simulink model "ICAR"  (R2018b)
settings: Solver=FixedStepAuto  StartTime=0.0  StopTime=10.0  RelTol=1e-3
(part 2 of 4)

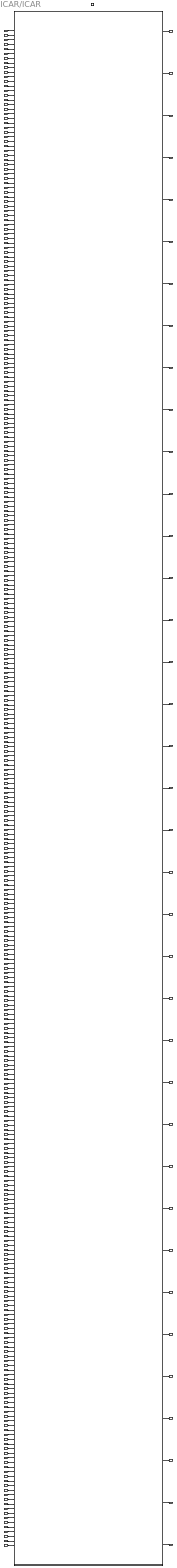
== system ICAR/ICAR ==
  System_Clock : Inport  OutDataTypeStr=UInt16
  FDMMve_d_IcaFcnConf : Inport  Port=2  OutDataTypeStr=UInt16
  FDMMve_d_SignalTStamp : Inport  Port=3  OutDataTypeStr=UInt16
  ICABva_g_VehParameter : Inport  Port=4  OutDataTypeStr=T_M_Nm_Float32  PortDimensions=60
  ICABva_g_FilterInfo : Inport  Port=5  OutDataTypeStr=T_M_Nm_Float32  PortDimensions=50
  ICABve_d_SignalTStamp : Inport  Port=6  OutDataTypeStr=UInt16
  IMAPve_d_EPS_LKA_State : Inport  Port=7  OutDataTypeStr=UInt16
  IMAPve_g_EPS_SW_Trq : Inport  Port=8  OutDataTypeStr=T_M_Nm_Float32
  IMAPve_d_EPS_Error_State : Inport  Port=9  OutDataTypeStr=UInt16
  IMAPve_d_EPS_Trq_State : Inport  Port=10  OutDataTypeStr=UInt16
  IMAPve_d_SAS_Clb_State : Inport  Port=11  OutDataTypeStr=UInt16
  IMAPve_d_SAS_Trim_State : Inport  Port=12  OutDataTypeStr=UInt16
  IMAPve_d_EPS_TrqLim_State : Inport  Port=13  OutDataTypeStr=UInt16
  IMAPve_g_EPS_LKA_Current : Inport  Port=14  OutDataTypeStr=T_M_Nm_Float32
  IMAPve_g_ESC_LatAcc : Inport  Port=15  OutDataTypeStr=T_M_Nm_Float32
  IMAPve_d_ESC_LatAcc_Valid : Inport  Port=16  OutDataTypeStr=UInt16
  IMAPve_g_ESC_YawRate : Inport  Port=17  OutDataTypeStr=T_M_Nm_Float32
  IMAPve_d_ESC_YawRate_Valid : Inport  Port=18  OutDataTypeStr=UInt16
  IMAPve_g_ESC_UnYawRate : Inport  Port=19  OutDataTypeStr=T_M_Nm_Float32
  IMAPve_g_ESC_VehSpd : Inport  Port=20  OutDataTypeStr=T_M_Nm_Float32
  IMAPve_g_ESC_LonAcc : Inport  Port=21  OutDataTypeStr=T_M_Nm_Float32
  IMAPve_d_ESC_LonAcc_Valid : Inport  Port=22  OutDataTypeStr=UInt16
  IMAPve_g_ESC_Brake_Press : Inport  Port=23  OutDataTypeStr=T_M_Nm_Float32
  IMAPve_g_ESC_Static_Slope : Inport  Port=24  OutDataTypeStr=T_M_Nm_Float32
  IMAPve_g_ESC_DySlope_Accuracy : Inport  Port=25  OutDataTypeStr=T_M_Nm_Float32
  IMAPve_g_ESC_DySlope : Inport  Port=26  OutDataTypeStr=T_M_Nm_Float32
  IMAPve_g_SW_Angle : Inport  Port=27  OutDataTypeStr=T_M_Nm_Float32
  IMAPve_g_SW_Angle_Speed : Inport  Port=28  OutDataTypeStr=T_M_Nm_Float32
  IMAPve_d_BCM_HazardLamp : Inport  Port=29  OutDataTypeStr=UInt16
  IMAPve_d_BCM_Left_Light : Inport  Port=30  OutDataTypeStr=UInt16
  IMAPve_d_BCM_Right_Light : Inport  Port=31  OutDataTypeStr=UInt16
  IMAPve_d_ESC_BrakeLamp_Req : Inport  Port=32  OutDataTypeStr=UInt16
  IMAPve_d_BCM_Opening_State : Inport  Port=33  OutDataTypeStr=UInt16
  IMAPve_d_BCM_Trunk_State : Inport  Port=34  OutDataTypeStr=UInt16
  IMAPve_d_BCM_LF_Door_State : Inport  Port=35  OutDataTypeStr=UInt16
  IMAPve_d_BCM_RF_Door_State : Inport  Port=36  OutDataTypeStr=UInt16
  IMAPve_d_BCM_RR_Door_State : Inport  Port=37  OutDataTypeStr=UInt16
  IMAPve_d_BCM_LR_Door_State : Inport  Port=38  OutDataTypeStr=UInt16
  IMAPve_d_SCC_Left_SwitchSig : Inport  Port=39  OutDataTypeStr=UInt16
  IMAPve_d_SCC_Right_SwitchSig : Inport  Port=40  OutDataTypeStr=UInt16
  IMAPve_d_PEPS_Door_Lock_Req : Inport  Port=41  OutDataTypeStr=UInt16
  IMAPve_d_BCM_Door_Lock_State : Inport  Port=42  OutDataTypeStr=UInt16
  IMAPve_d_EMS_ACC_Status : Inport  Port=43  OutDataTypeStr=UInt16
  IMAPve_g_EMS_Pot_WhlT_Max : Inport  Port=44  OutDataTypeStr=T_M_Nm_Float32
  IMAPve_g_EMS_Pot_WhlT_Min : Inport  Port=45  OutDataTypeStr=T_M_Nm_Float32
  IMAPve_g_EMS_RealPedal : Inport  Port=46  OutDataTypeStr=T_M_Nm_Float32
  IMAPve_g_EMS_MaxTWhl : Inport  Port=47  OutDataTypeStr=T_M_Nm_Float32
  IMAPve_g_EMS_MaxTWhl_Offset : Inport  Port=48  OutDataTypeStr=T_M_Nm_Float32
  IMAPve_g_EMS_MinTWhl : Inport  Port=49  OutDataTypeStr=T_M_Nm_Float32
  IMAPve_g_EMS_MinTWhl_Offset : Inport  Port=50  OutDataTypeStr=T_M_Nm_Float32
  IMAPve_g_EMS_Actual_FlwT : Inport  Port=51  OutDataTypeStr=T_M_Nm_Float32
  IMAPve_g_EMS_Actual_IndT : Inport  Port=52  OutDataTypeStr=T_M_Nm_Float32
  IMAPve_g_EMS_Realize_TWhl : Inport  Port=53  OutDataTypeStr=T_M_Nm_Float32
  IMAPve_g_EMS_ACC_VirtualPedal : Inport  Port=54  OutDataTypeStr=T_M_Nm_Float32
  IMAPve_d_EMS_AccPedal_Fault : Inport  Port=55  OutDataTypeStr=UInt16
  IMAPve_g_EMS_Driver_Torque : Inport  Port=56  OutDataTypeStr=T_M_Nm_Float32
  IMAPve_d_ESC_Brake_Effort : Inport  Port=57  OutDataTypeStr=UInt16
  IMAPve_g_EMS_Engine_Speed : Inport  Port=58  OutDataTypeStr=T_M_Nm_Float32
  IMAPve_d_ESC_Veh_Standstill : Inport  Port=59  OutDataTypeStr=UInt16
  IMAPve_d_TCU_Actual_Gear : Inport  Port=60  OutDataTypeStr=UInt16
  IMAPve_d_TCU_Target_Gear : Inport  Port=61  OutDataTypeStr=UInt16
  IMAPve_d_TCU_PRND_State : Inport  Port=62  OutDataTypeStr=UInt16
  IMAPve_d_BCM_Ignition_State : Inport  Port=63  OutDataTypeStr=UInt16
  IMAPve_d_ACU_Driver_Belt : Inport  Port=64  OutDataTypeStr=UInt16
  IMAPve_d_SWS_Fault_Code : Inport  Port=65  OutDataTypeStr=UInt16
  IMAPve_d_SWS_Failure_Status : Inport  Port=66  OutDataTypeStr=UInt16
  IMAPve_d_ESC_OFF : Inport  Port=67  OutDataTypeStr=UInt16
  IMAPve_d_ESC_AlarmSig : Inport  Port=68  OutDataTypeStr=UInt16
  IMAPve_d_Speed_Limit_Switch : Inport  Port=69  OutDataTypeStr=UInt16
  IMAPve_d_ESC_ESC_Active : Inport  Port=70  OutDataTypeStr=UInt16
  IMAPve_d_ESC_MSR_Active : Inport  Port=71  OutDataTypeStr=UInt16
  IMAPve_d_ESC_TCS_Active : Inport  Port=72  OutDataTypeStr=UInt16
  IMAPve_d_ESC_VehSpd_Valid : Inport  Port=73  OutDataTypeStr=UInt16
  IMAPve_d_Brake_Pedal_Fault : Inport  Port=74  OutDataTypeStr=UInt16
  IMAPve_d_ESC_ABS_Active : Inport  Port=75  OutDataTypeStr=UInt16
  IMAPve_d_ESC_ABS_Valid : Inport  Port=76  OutDataTypeStr=UInt16
  IMAPve_d_ESC_ABS_AlarmSig : Inport  Port=77  OutDataTypeStr=UInt16
  IMAPve_d_ESC_FL_WheelPulVal : Inport  Port=78  OutDataTypeStr=UInt16
  IMAPve_d_ESC_FR_WheelPulVal : Inport  Port=79  OutDataTypeStr=UInt16
  IMAPve_d_ESC_RL_WheelPulVal : Inport  Port=80  OutDataTypeStr=UInt16
  IMAPve_d_ESC_RR_WheelPulVal : Inport  Port=81  OutDataTypeStr=UInt16
  IMAPve_g_ESC_FL_WhlSpd : Inport  Port=82  OutDataTypeStr=T_M_Nm_Float32
  IMAPve_d_ESC_FL_WhlSpd_Fault : Inport  Port=83  OutDataTypeStr=UInt16
  IMAPve_g_ESC_FR_WhlSpd : Inport  Port=84  OutDataTypeStr=T_M_Nm_Float32
  IMAPve_d_ESC_FR_WhlSpd_Fault : Inport  Port=85  OutDataTypeStr=UInt16
  IMAPve_g_ESC_RL_WhlSpd : Inport  Port=86  OutDataTypeStr=T_M_Nm_Float32
  IMAPve_d_ESC_RL_WhlSpd_Fault : Inport  Port=87  OutDataTypeStr=UInt16
  IMAPve_g_ESC_RR_WhlSpd : Inport  Port=88  OutDataTypeStr=T_M_Nm_Float32
  IMAPve_d_ESC_RR_WhlSpd_Fault : Inport  Port=89  OutDataTypeStr=UInt16
  IMAPve_d_ESC_FL_Wheel_Pulse : Inport  Port=90  OutDataTypeStr=UInt16
  IMAPve_d_ESC_FR_Wheel_Pulse : Inport  Port=91  OutDataTypeStr=UInt16
  IMAPve_d_ESC_RL_Wheel_Pulse : Inport  Port=92  OutDataTypeStr=UInt16
  IMAPve_d_ESC_RR_Wheel_Pulse : Inport  Port=93  OutDataTypeStr=UInt16
  IMAPve_d_TCU_AT_Failure : Inport  Port=94  OutDataTypeStr=UInt16
  IMAPve_d_TCU_Shift_Valid : Inport  Port=95  OutDataTypeStr=UInt16
  IMAPve_d_TCU_DCT_Clutch_State : Inport  Port=96  OutDataTypeStr=UInt16
  IMAPve_d_TCU_Gear_Engage : Inport  Port=97  OutDataTypeStr=UInt16
  IMAPve_d_TCU_Select_ATMode : Inport  Port=98  OutDataTypeStr=UInt16
  IMAPve_d_EMS_Engine_Status : Inport  Port=99  OutDataTypeStr=UInt16
  IMAPve_d_EMS_Gearbox_CtlAvail : Inport  Port=100  OutDataTypeStr=UInt16
  IMAPve_d_ESC_Brake_Failsafe : Inport  Port=101  OutDataTypeStr=UInt16
  IMAPve_d_ESC_AEB_Status : Inport  Port=102  OutDataTypeStr=UInt16
  IMAPve_d_ESC_AEB_Available : Inport  Port=103  OutDataTypeStr=UInt16
  IMAPve_d_ESC_AEB_Active : Inport  Port=104  OutDataTypeStr=UInt16
  IMAPve_d_ESC_ACC_Status : Inport  Port=105  OutDataTypeStr=UInt16
  IMAPve_d_ESC_ACC_Available : Inport  Port=106  OutDataTypeStr=UInt16
  IMAPve_d_ESC_ACC_Active : Inport  Port=107  OutDataTypeStr=UInt16
  IMAPve_d_EMS_ACC_Effective : Inport  Port=108  OutDataTypeStr=UInt16
  IMAPve_d_BCM_FrontWiper_State : Inport  Port=109  OutDataTypeStr=UInt16
  IMAPve_d_BCM_CHMSL_Status : Inport  Port=110  OutDataTypeStr=UInt16
  IMAPve_d_BCM_BrakeLamp_State : Inport  Port=111  OutDataTypeStr=UInt16
  IMAPve_d_GW_Brake_Only_Req : Inport  Port=112  OutDataTypeStr=UInt16
  IMAPve_d_ACU_Passenger_Belt : Inport  Port=113  OutDataTypeStr=UInt16
  IMAPve_d_EMS_ACC_CtlAvail : Inport  Port=114  OutDataTypeStr=UInt16
  IMAPve_d_EMS_ACC_Inhibited : Inport  Port=115  OutDataTypeStr=UInt16
  IMAPve_d_EMS_Brake_Pedal : Inport  Port=116  OutDataTypeStr=UInt16
  IMAPve_d_BCM_LowBeam_State : Inport  Port=117  OutDataTypeStr=UInt16
  IMAPve_d_BCM_HighBeam_State : Inport  Port=118  OutDataTypeStr=UInt16
  IMAPve_d_EPB_Status : Inport  Port=119  OutDataTypeStr=UInt16
  IMAPve_d_EPB_Display_Req : Inport  Port=120  OutDataTypeStr=UInt16
  IMAPve_d_EPB_Warn_Req : Inport  Port=121  OutDataTypeStr=UInt16
  IMAPve_d_EPB_Switch_State : Inport  Port=122  OutDataTypeStr=UInt16
  IMAPve_d_EPB_Switch_Valid : Inport  Port=123  OutDataTypeStr=UInt16
  IMAPve_d_ESC_Drive_Direction : Inport  Port=124  OutDataTypeStr=UInt16
  IMAPve_d_ESC_Hold_State : Inport  Port=125  OutDataTypeStr=UInt16
  IMAPve_d_EPS_Steer_Hold_State : Inport  Port=126  OutDataTypeStr=UInt16
  IMAPve_d_EPS_Warning_State : Inport  Port=127  OutDataTypeStr=UInt16
  IMAPve_g_EPS_PowerCon : Inport  Port=128  OutDataTypeStr=T_M_Nm_Float32
  IMAPve_d_ESC_EBD_AlarmSig : Inport  Port=129  OutDataTypeStr=UInt16
  IMAPve_d_ESC_AVH_Status : Inport  Port=130  OutDataTypeStr=UInt16
  IMAPve_d_Radar_Detective_Req : Inport  Port=131  OutDataTypeStr=UInt16
  IMAPve_g_BCM_Battery_Voltage : Inport  Port=132  OutDataTypeStr=T_M_Nm_Float32
  IMAPve_d_TBOX_LocalTimeY : Inport  Port=133  OutDataTypeStr=UInt16
  IMAPve_d_TBOX_LocalTimeM : Inport  Port=134  OutDataTypeStr=UInt16
  IMAPve_d_TBOX_LocalTimeD : Inport  Port=135  OutDataTypeStr=UInt16
  IMAPve_d_TBOX_LocalTimeH : Inport  Port=136  OutDataTypeStr=UInt16
  IMAPve_d_TBOX_LocalTimeMin : Inport  Port=137  OutDataTypeStr=UInt16
  IMAPve_d_TBOX_LocalTimeS : Inport  Port=138  OutDataTypeStr=UInt16
  IMAPve_d_TBOX_LocalTime_Valid : Inport  Port=139  OutDataTypeStr=UInt16
  IMAPve_d_TPMS_Warn_Indicate : Inport  Port=140  OutDataTypeStr=UInt16
  IMAPve_d_Radar_State : Inport  Port=141  OutDataTypeStr=UInt16
  IMAPve_d_ACC_Desired_Headway : Inport  Port=142  OutDataTypeStr=UInt16
  IMAPve_d_Time_System_Clock : Inport  Port=143  OutDataTypeStr=UInt16
  IMAPve_d_Signal_Time_Stamp : Inport  Port=144  OutDataTypeStr=UInt16
  IMAPve_g_GW_IC_Odometer : Inport  Port=145  OutDataTypeStr=UInt32
  IMAPve_g_FAPA_State : Inport  Port=146  OutDataTypeStr=UInt32
  IMAPve_d_Outside_Temp : Inport  Port=147  OutDataTypeStr=UInt16
  IMAPve_d_ORI_CIPV_ID : Inport  Port=148  OutDataTypeStr=UInt16
  IMAPve_d_ORI_Obj_Num : Inport  Port=149  OutDataTypeStr=UInt16
  IMAPva_g_ORI_Probability : Inport  Port=150  OutDataTypeStr=T_M_Nm_Float32  PortDimensions=16
  IMAPva_d_ORI_Obj_Class : Inport  Port=151  OutDataTypeStr=UInt16  PortDimensions=16
  IMAPva_d_ORI_Obj_Motion : Inport  Port=152  OutDataTypeStr=UInt16  PortDimensions=16
  IMAPva_g_ORI_Obj_RelVel : Inport  Port=153  OutDataTypeStr=T_M_Nm_Float32  PortDimensions=16
  IMAPva_g_ORI_Obj_LongDis : Inport  Port=154  OutDataTypeStr=T_M_Nm_Float32  PortDimensions=16
  IMAPva_d_ORI_Obj_Lane : Inport  Port=155  OutDataTypeStr=UInt16  PortDimensions=16
  IMAPva_g_ORI_Obj_LAngle : Inport  Port=156  OutDataTypeStr=T_M_Nm_Float32  PortDimensions=16
  IMAPva_g_ORI_Obj_RAngle : Inport  Port=157  OutDataTypeStr=T_M_Nm_Float32  PortDimensions=16
  IMAPva_g_ORI_Obj_Width : Inport  Port=158  OutDataTypeStr=T_M_Nm_Float32  PortDimensions=16
  IMAPva_d_ORI_Obj_ID : Inport  Port=159  OutDataTypeStr=UInt16  PortDimensions=16
  IMAPve_d_ORI_Lane_Valid : Inport  Port=160  OutDataTypeStr=UInt16
  IMAPve_d_ORI_Lane_ConsArea : Inport  Port=161  OutDataTypeStr=UInt16
  IMAPve_d_ORI_Lane_RoadType : Inport  Port=162  OutDataTypeStr=UInt16
  IMAPve_g_ORI_L0_C3 : Inport  Port=163  OutDataTypeStr=T_M_Nm_Float32
  IMAPve_g_ORI_L0_C2 : Inport  Port=164  OutDataTypeStr=T_M_Nm_Float32
  IMAPve_g_ORI_L0_C1 : Inport  Port=165  OutDataTypeStr=T_M_Nm_Float32
  IMAPve_g_ORI_L0_C0 : Inport  Port=166  OutDataTypeStr=T_M_Nm_Float32
  IMAPve_d_ORI_L0_Q : Inport  Port=167  OutDataTypeStr=UInt16
  IMAPve_d_ORI_L0_Type : Inport  Port=168  OutDataTypeStr=UInt16
  IMAPve_g_ORI_L0_VR : Inport  Port=169  OutDataTypeStr=T_M_Nm_Float32
  IMAPve_g_ORI_L0_TLC : Inport  Port=170  OutDataTypeStr=T_M_Nm_Float32
  IMAPve_g_ORI_L0_W : Inport  Port=171  OutDataTypeStr=T_M_Nm_Float32
  IMAPve_d_ORI_L0_LC : Inport  Port=172  OutDataTypeStr=UInt16
  IMAPve_g_ORI_L1_C3 : Inport  Port=173  OutDataTypeStr=T_M_Nm_Float32
  IMAPve_g_ORI_L1_C2 : Inport  Port=174  OutDataTypeStr=T_M_Nm_Float32
  IMAPve_g_ORI_L1_C1 : Inport  Port=175  OutDataTypeStr=T_M_Nm_Float32
  IMAPve_g_ORI_L1_C0 : Inport  Port=176  OutDataTypeStr=T_M_Nm_Float32
  IMAPve_d_ORI_L1_Q : Inport  Port=177  OutDataTypeStr=UInt16
  IMAPve_d_ORI_L1_Type : Inport  Port=178  OutDataTypeStr=UInt16
  IMAPve_g_ORI_L1_VR : Inport  Port=179  OutDataTypeStr=T_M_Nm_Float32
  IMAPve_g_ORI_L1_TLC : Inport  Port=180  OutDataTypeStr=T_M_Nm_Float32
  IMAPve_g_ORI_L1_W : Inport  Port=181  OutDataTypeStr=T_M_Nm_Float32
  IMAPve_d_ORI_L1_LC : Inport  Port=182  OutDataTypeStr=UInt16
  IMAPve_g_ORI_R0_C3 : Inport  Port=183  OutDataTypeStr=T_M_Nm_Float32
  IMAPve_g_ORI_R0_C2 : Inport  Port=184  OutDataTypeStr=T_M_Nm_Float32
  IMAPve_g_ORI_R0_C1 : Inport  Port=185  OutDataTypeStr=T_M_Nm_Float32
  IMAPve_g_ORI_R0_C0 : Inport  Port=186  OutDataTypeStr=T_M_Nm_Float32
  IMAPve_d_ORI_R0_Q : Inport  Port=187  OutDataTypeStr=UInt16
  IMAPve_d_ORI_R0_LT : Inport  Port=188  OutDataTypeStr=UInt16
  IMAPve_g_ORI_R0_VR : Inport  Port=189  OutDataTypeStr=T_M_Nm_Float32
  IMAPve_g_ORI_R0_TLC : Inport  Port=190  OutDataTypeStr=T_M_Nm_Float32
  IMAPve_g_ORI_R0_W : Inport  Port=191  OutDataTypeStr=T_M_Nm_Float32
  IMAPve_d_ORI_R0_LC : Inport  Port=192  OutDataTypeStr=UInt16
  IMAPve_g_ORI_R1_C3 : Inport  Port=193  OutDataTypeStr=T_M_Nm_Float32
  IMAPve_g_ORI_R1_C2 : Inport  Port=194  OutDataTypeStr=T_M_Nm_Float32
  IMAPve_g_ORI_R1_C1 : Inport  Port=195  OutDataTypeStr=T_M_Nm_Float32
  IMAPve_g_ORI_R1_C0 : Inport  Port=196  OutDataTypeStr=T_M_Nm_Float32
  IMAPve_d_ORI_R1_Q : Inport  Port=197  OutDataTypeStr=UInt16
  IMAPve_d_ORI_R1_LT : Inport  Port=198  OutDataTypeStr=UInt16
  IMAPve_g_ORI_R1_VR : Inport  Port=199  OutDataTypeStr=T_M_Nm_Float32
  IMAPve_g_ORI_R1_TLC : Inport  Port=200  OutDataTypeStr=T_M_Nm_Float32
  IMAPve_g_ORI_R1_W : Inport  Port=201  OutDataTypeStr=T_M_Nm_Float32
  IMAPve_d_ORI_R1_LC : Inport  Port=202  OutDataTypeStr=UInt16
  IMAPve_d_Sensor_Status : Inport  Port=203  OutDataTypeStr=UInt16
  IMAPve_d_LF_Radar_Status : Inport  Port=204  OutDataTypeStr=UInt16
  IMAPve_d_RF_Radar_Status : Inport  Port=205  OutDataTypeStr=UInt16
  IMAPve_d_LR_Radar_Status : Inport  Port=206  OutDataTypeStr=UInt16
  IMAPve_d_RR_Radar_Status : Inport  Port=207  OutDataTypeStr=UInt16
  IMAPve_d_Fusion_Status : Inport  Port=208  OutDataTypeStr=UInt16
  IMAPve_g_Fusion_Time_Stamp : Inport  Port=209  OutDataTypeStr=T_M_Nm_Float32
  IMAPve_d_obj_Num : Inport  Port=210  OutDataTypeStr=UInt16
  IMAPva_d_obj_id : Inport  Port=211  OutDataTypeStr=UInt16  PortDimensions=40
  IMAPva_g_obj_pos_x : Inport  Port=212  OutDataTypeStr=T_M_Nm_Float32  PortDimensions=40
  IMAPva_g_obj_pos_y : Inport  Port=213  OutDataTypeStr=T_M_Nm_Float32  PortDimensions=40
  IMAPva_g_obj_vel_x : Inport  Port=214  OutDataTypeStr=T_M_Nm_Float32  PortDimensions=40
  IMAPva_g_obj_vel_y : Inport  Port=215  OutDataTypeStr=T_M_Nm_Float32  PortDimensions=40
  IMAPva_g_obj_acc_x : Inport  Port=216  OutDataTypeStr=T_M_Nm_Float32  PortDimensions=40
  IMAPva_g_obj_acc_y : Inport  Port=217  OutDataTypeStr=T_M_Nm_Float32  PortDimensions=40
  IMAPva_g_obj_pos_var_x : Inport  Port=218  OutDataTypeStr=T_M_Nm_Float32  PortDimensions=40
  IMAPva_g_obj_pos_var_y : Inport  Port=219  OutDataTypeStr=T_M_Nm_Float32  PortDimensions=40
  IMAPva_g_obj_pos_var_xy : Inport  Port=220  OutDataTypeStr=T_M_Nm_Float32  PortDimensions=40
  IMAPva_g_obj_vel_var_x : Inport  Port=221  OutDataTypeStr=T_M_Nm_Float32  PortDimensions=40
  IMAPva_g_obj_vel_var_y : Inport  Port=222  OutDataTypeStr=T_M_Nm_Float32  PortDimensions=40
  IMAPva_g_obj_vel_var_xy : Inport  Port=223  OutDataTypeStr=T_M_Nm_Float32  PortDimensions=40
  IMAPva_g_obj_width : Inport  Port=224  OutDataTypeStr=T_M_Nm_Float32  PortDimensions=40
  IMAPva_g_obj_length : Inport  Port=225  OutDataTypeStr=T_M_Nm_Float32  PortDimensions=40
  IMAPva_d_obj_fusion_type : Inport  Port=226  OutDataTypeStr=UInt16  PortDimensions=40
  IMAPva_d_obj_class : Inport  Port=227  OutDataTypeStr=UInt16  PortDimensions=40
  IMAPva_d_obj_lane : Inport  Port=228  OutDataTypeStr=UInt16  PortDimensions=40
  IMAPva_d_obj_status : Inport  Port=229  OutDataTypeStr=UInt16  PortDimensions=40
  IMAPva_d_obj_cam_asso_id : Inport  Port=230  OutDataTypeStr=UInt16  PortDimensions=40
  IMAPva_g_obj_con : Inport  Port=231  OutDataTypeStr=T_M_Nm_Float32  PortDimensions=40
  IMAPva_g_obj_age : Inport  Port=232  OutDataTypeStr=T_M_Nm_Float32  PortDimensions=40
  IMAPva_d_obj_TurnLight : Inport  Port=233  OutDataTypeStr=UInt16  PortDimensions=40
  IMAPva_d_obj_BrakeLight : Inport  Port=234  OutDataTypeStr=UInt16  PortDimensions=40
  IMAPva_d_obj_MotionStatus : Inport  Port=235  OutDataTypeStr=UInt16  PortDimensions=40
  IMAPva_d_obj_ACC : Inport  Port=236  OutDataTypeStr=UInt16  PortDimensions=40
  IMAPva_d_obj_AEB : Inport  Port=237  OutDataTypeStr=UInt16  PortDimensions=40
  IMAPva_d_obj_ELK : Inport  Port=238  OutDataTypeStr=UInt16  PortDimensions=40
  IMAPva_d_obj_ALC : Inport  Port=239  OutDataTypeStr=UInt16  PortDimensions=40
  IMAPva_d_obj_ESA : Inport  Port=240  OutDataTypeStr=UInt16  PortDimensions=40
  IMAPva_d_obj_JA : Inport  Port=241  OutDataTypeStr=UInt16  PortDimensions=40
  IMAPve_d_Lane_Valid : Inport  Port=242  OutDataTypeStr=UInt16
  IMAPve_d_Road_Type : Inport  Port=243  OutDataTypeStr=UInt16
  IMAPve_d_ConsArea : Inport  Port=244  OutDataTypeStr=UInt16
  IMAPve_g_L0_C0 : Inport  Port=245  OutDataTypeStr=T_M_Nm_Float32
  IMAPve_g_L0_C1 : Inport  Port=246  OutDataTypeStr=T_M_Nm_Float32
  IMAPve_g_L0_C2 : Inport  Port=247  OutDataTypeStr=T_M_Nm_Float32
  IMAPve_g_L0_C3 : Inport  Port=248  OutDataTypeStr=T_M_Nm_Float32
  IMAPve_g_L0_VR : Inport  Port=249  OutDataTypeStr=T_M_Nm_Float32
  IMAPve_d_L0_Q : Inport  Port=250  OutDataTypeStr=UInt16
  IMAPve_d_L0_Type : Inport  Port=251  OutDataTypeStr=UInt16
  IMAPve_g_L0_Confidence : Inport  Port=252  OutDataTypeStr=T_M_Nm_Float32
  IMAPve_g_L0_W : Inport  Port=253  OutDataTypeStr=T_M_Nm_Float32
  IMAPve_g_L0_TLC : Inport  Port=254  OutDataTypeStr=T_M_Nm_Float32
  IMAPve_d_L0_LC : Inport  Port=255  OutDataTypeStr=UInt16
  IMAPve_g_R0_C0 : Inport  Port=256  OutDataTypeStr=T_M_Nm_Float32
  IMAPve_g_R0_C1 : Inport  Port=257  OutDataTypeStr=T_M_Nm_Float32
  IMAPve_g_R0_C2 : Inport  Port=258  OutDataTypeStr=T_M_Nm_Float32
  IMAPve_g_R0_C3 : Inport  Port=259  OutDataTypeStr=T_M_Nm_Float32
  IMAPve_g_R0_VR : Inport  Port=260  OutDataTypeStr=T_M_Nm_Float32
  IMAPve_d_R0_Q : Inport  Port=261  OutDataTypeStr=UInt16
  IMAPve_d_R0_Type : Inport  Port=262  OutDataTypeStr=UInt16
  IMAPve_g_R0_Confidence : Inport  Port=263  OutDataTypeStr=T_M_Nm_Float32
  IMAPve_g_R0_W : Inport  Port=264  OutDataTypeStr=T_M_Nm_Float32
  IMAPve_g_R0_TLC : Inport  Port=265  OutDataTypeStr=T_M_Nm_Float32
  IMAPve_d_R0_LC : Inport  Port=266  OutDataTypeStr=UInt16
  IMAPve_g_L1_C0 : Inport  Port=267  OutDataTypeStr=T_M_Nm_Float32
  IMAPve_g_L1_C1 : Inport  Port=268  OutDataTypeStr=T_M_Nm_Float32
  IMAPve_g_L1_C2 : Inport  Port=269  OutDataTypeStr=T_M_Nm_Float32
  IMAPve_g_L1_C3 : Inport  Port=270  OutDataTypeStr=T_M_Nm_Float32
  IMAPve_g_L1_VR : Inport  Port=271  OutDataTypeStr=T_M_Nm_Float32
  IMAPve_d_L1_Q : Inport  Port=272  OutDataTypeStr=UInt16
  IMAPve_d_L1_Type : Inport  Port=273  OutDataTypeStr=UInt16
  IMAPve_g_L1_Confidence : Inport  Port=274  OutDataTypeStr=T_M_Nm_Float32
  IMAPve_g_L1_W : Inport  Port=275  OutDataTypeStr=T_M_Nm_Float32
  IMAPve_g_L1_TLC : Inport  Port=276  OutDataTypeStr=T_M_Nm_Float32
  IMAPve_d_L1_LC : Inport  Port=277  OutDataTypeStr=UInt16
  IMAPve_g_R1_C0 : Inport  Port=278  OutDataTypeStr=T_M_Nm_Float32
  IMAPve_g_R1_C1 : Inport  Port=279  OutDataTypeStr=T_M_Nm_Float32
  IMAPve_g_R1_C2 : Inport  Port=280  OutDataTypeStr=T_M_Nm_Float32
  IMAPve_g_R1_C3 : Inport  Port=281  OutDataTypeStr=T_M_Nm_Float32
  IMAPve_g_R1_VR : Inport  Port=282  OutDataTypeStr=T_M_Nm_Float32
  IMAPve_d_R1_Q : Inport  Port=283  OutDataTypeStr=UInt16
  IMAPve_d_R1_Type : Inport  Port=284  OutDataTypeStr=UInt16
  IMAPve_g_R1_Confidence : Inport  Port=285  OutDataTypeStr=T_M_Nm_Float32
  IMAPve_g_R1_W : Inport  Port=286  OutDataTypeStr=T_M_Nm_Float32
  IMAPve_g_R1_TLC : Inport  Port=287  OutDataTypeStr=T_M_Nm_Float32
  IMAPve_d_R1_LC : Inport  Port=288  OutDataTypeStr=UInt16
  IMAPve_g_L0_C0_Back : Inport  Port=289  OutDataTypeStr=T_M_Nm_Float32
  IMAPve_g_L0_C1_Back : Inport  Port=290  OutDataTypeStr=T_M_Nm_Float32
  IMAPve_g_L0_C2_Back : Inport  Port=291  OutDataTypeStr=T_M_Nm_Float32
  IMAPve_g_L0_C3_Back : Inport  Port=292  OutDataTypeStr=T_M_Nm_Float32
  IMAPve_g_L0_Range_Back : Inport  Port=293  OutDataTypeStr=T_M_Nm_Float32
  IMAPve_g_L0_C0_FR_Pred : Inport  Port=294  OutDataTypeStr=T_M_Nm_Float32
  IMAPve_g_L0_C1_FR_Pred : Inport  Port=295  OutDataTypeStr=T_M_Nm_Float32
  IMAPve_g_L0_C2_FR_Pred : Inport  Port=296  OutDataTypeStr=T_M_Nm_Float32
  IMAPve_g_L0_Range_FR_Pred : Inport  Port=297  OutDataTypeStr=T_M_Nm_Float32
  IMAPve_g_R0_C0_Back : Inport  Port=298  OutDataTypeStr=T_M_Nm_Float32
  IMAPve_g_R0_C1_Back : Inport  Port=299  OutDataTypeStr=T_M_Nm_Float32
  IMAPve_g_R0_C2_Back : Inport  Port=300  OutDataTypeStr=T_M_Nm_Float32
  IMAPve_g_R0_C3_Back : Inport  Port=301  OutDataTypeStr=T_M_Nm_Float32
  IMAPve_g_R0_Range_Back : Inport  Port=302  OutDataTypeStr=T_M_Nm_Float32
  IMAPve_g_R0_C0_FR_Pred : Inport  Port=303  OutDataTypeStr=T_M_Nm_Float32
  IMAPve_g_R0_C1_FR_Pred : Inport  Port=304  OutDataTypeStr=T_M_Nm_Float32
  IMAPve_g_R0_C2_FR_Pred : Inport  Port=305  OutDataTypeStr=T_M_Nm_Float32
  IMAPve_g_R0_Range_FR_Pred : Inport  Port=306  OutDataTypeStr=T_M_Nm_Float32
  IMAPve_g_L1_C0_Back : Inport  Port=307  OutDataTypeStr=T_M_Nm_Float32
  IMAPve_g_L1_C1_Back : Inport  Port=308  OutDataTypeStr=T_M_Nm_Float32
  IMAPve_g_L1_C2_Back : Inport  Port=309  OutDataTypeStr=T_M_Nm_Float32
  IMAPve_g_L1_C3_Back : Inport  Port=310  OutDataTypeStr=T_M_Nm_Float32
  IMAPve_g_L1_Range_Back : Inport  Port=311  OutDataTypeStr=T_M_Nm_Float32
  IMAPve_g_L1_C0_FR_Pred : Inport  Port=312  OutDataTypeStr=T_M_Nm_Float32
  IMAPve_g_L1_C1_FR_Pred : Inport  Port=313  OutDataTypeStr=T_M_Nm_Float32
  IMAPve_g_L1_C2_FR_Pred : Inport  Port=314  OutDataTypeStr=T_M_Nm_Float32
  IMAPve_g_L1_Range_FR_Pred : Inport  Port=315  OutDataTypeStr=T_M_Nm_Float32
  IMAPve_g_R1_C0_Back : Inport  Port=316  OutDataTypeStr=T_M_Nm_Float32
  IMAPve_g_R1_C1_Back : Inport  Port=317  OutDataTypeStr=T_M_Nm_Float32
  IMAPve_g_R1_C2_Back : Inport  Port=318  OutDataTypeStr=T_M_Nm_Float32
  IMAPve_g_R1_C3_Back : Inport  Port=319  OutDataTypeStr=T_M_Nm_Float32
  IMAPve_g_R1_Range_Back : Inport  Port=320  OutDataTypeStr=T_M_Nm_Float32
  IMAPve_g_R1_C0_FR_Pred : Inport  Port=321  OutDataTypeStr=T_M_Nm_Float32
  IMAPve_g_R1_C1_FR_Pred : Inport  Port=322  OutDataTypeStr=T_M_Nm_Float32
  IMAPve_g_R1_C2_FR_Pred : Inport  Port=323  OutDataTypeStr=T_M_Nm_Float32
  IMAPve_g_R1_Range_FR_Pred : Inport  Port=324  OutDataTypeStr=T_M_Nm_Float32
  IMAPve_d_Sign_ISA_Value : Inport  Port=325  OutDataTypeStr=UInt16
  IMAPve_d_TSR_Sign_Type : Inport  Port=326  OutDataTypeStr=UInt16
  IMAPve_d_Camera_Signal_Fault : Inport  Port=327  OutDataTypeStr=UInt16
  IMAPve_d_Radar_Status : Inport  Port=328  OutDataTypeStr=UInt16
  IMAPve_d_Camera_Status : Inport  Port=329  OutDataTypeStr=UInt16
  function : TriggerPort  TriggerType=function-call  VariantControl=Variant  SampleTimeType=periodic  SampleTime=-1
  ICAR : Subsystem  TreatAsAtomicUnit=on
  ICARva_d_obj_Num : Outport  OutDataTypeStr=UInt16  PortDimensions=40
  ICARva_d_obj_id : Outport  Port=2  OutDataTypeStr=UInt16  PortDimensions=40
  ICARva_g_obj_pos_x : Outport  Port=3  OutDataTypeStr=T_M_Nm_Float32  PortDimensions=40
  ICARva_g_obj_pos_y : Outport  Port=4  OutDataTypeStr=T_M_Nm_Float32  PortDimensions=40
  ICARva_g_obj_vel_x : Outport  Port=5  OutDataTypeStr=T_M_Nm_Float32  PortDimensions=40
  ICARva_g_obj_vel_y : Outport  Port=6  OutDataTypeStr=T_M_Nm_Float32  PortDimensions=40
  ICARva_g_obj_acc_x : Outport  Port=7  OutDataTypeStr=T_M_Nm_Float32  PortDimensions=40
  ICARva_g_obj_acc_y : Outport  Port=8  OutDataTypeStr=T_M_Nm_Float32  PortDimensions=40
  ICARva_g_obj_pos_var_x : Outport  Port=9  OutDataTypeStr=T_M_Nm_Float32  PortDimensions=40
  ICARva_g_obj_pos_var_y : Outport  Port=10  OutDataTypeStr=T_M_Nm_Float32  PortDimensions=40
  ICARva_g_obj_pos_var_xy : Outport  Port=11  OutDataTypeStr=T_M_Nm_Float32  PortDimensions=40
  ICARva_g_obj_vel_var_x : Outport  Port=12  OutDataTypeStr=T_M_Nm_Float32  PortDimensions=40
  ICARva_g_obj_vel_var_y : Outport  Port=13  OutDataTypeStr=T_M_Nm_Float32  PortDimensions=40
  ICARva_g_obj_vel_var_xy : Outport  Port=14  OutDataTypeStr=T_M_Nm_Float32  PortDimensions=40
  ICARva_g_obj_width : Outport  Port=15  OutDataTypeStr=T_M_Nm_Float32  PortDimensions=40
  ICARva_d_obj_length : Outport  Port=16  OutDataTypeStr=T_M_Nm_Float32  PortDimensions=40
  ICARva_d_obj_fusion_type : Outport  Port=17  OutDataTypeStr=UInt16  PortDimensions=40
  ICARva_d_obj_class : Outport  Port=18  OutDataTypeStr=UInt16  PortDimensions=40
  ICARva_d_obj_lane : Outport  Port=19  OutDataTypeStr=UInt16  PortDimensions=40
  ICARva_d_obj_status : Outport  Port=20  OutDataTypeStr=UInt16  PortDimensions=40
  ICARve_d_obj_cam_asso_id : Outport  Port=21  OutDataTypeStr=UInt16
  ICARva_g_obj_con : Outport  Port=22  OutDataTypeStr=T_M_Nm_Float32  PortDimensions=40
  ICARva_d_obj_age : Outport  Port=23  OutDataTypeStr=UInt16  PortDimensions=40
  ICARva_d_obj_TurnLight : Outport  Port=24  OutDataTypeStr=UInt16  PortDimensions=40
  ICARva_d_obj_BrakeLight : Outport  Port=25  OutDataTypeStr=UInt16  PortDimensions=40
  ICARva_d_obj_MotionStatus : Outport  Port=26  OutDataTypeStr=UInt16  PortDimensions=40
  ICARva_g_ObjXPre : Outport  Port=27  OutDataTypeStr=T_M_Nm_Float32  PortDimensions=240
  ICARva_g_ObjYPre : Outport  Port=28  OutDataTypeStr=T_M_Nm_Float32  PortDimensions=240
  ICARva_g_ObjVarXPre : Outport  Port=29  OutDataTypeStr=T_M_Nm_Float32  PortDimensions=240
  ICARva_g_ObjVarYPre : Outport  Port=30  OutDataTypeStr=T_M_Nm_Float32  PortDimensions=240
  ICARva_g_ObjVarXYPre : Outport  Port=31  OutDataTypeStr=T_M_Nm_Float32  PortDimensions=240
  ICARva_g_ObjVelXPre : Outport  Port=32  OutDataTypeStr=T_M_Nm_Float32  PortDimensions=240
  ICARva_g_ObjVelYPre : Outport  Port=33  OutDataTypeStr=T_M_Nm_Float32  PortDimensions=240
  ICARva_g_ObjVelVarXPre : Outport  Port=34  OutDataTypeStr=T_M_Nm_Float32  PortDimensions=240
  ICARva_g_ObjVelVarYPre : Outport  Port=35  OutDataTypeStr=T_M_Nm_Float32  PortDimensions=240
  ICARva_g_ObjVelVarXYPre : Outport  Port=36  OutDataTypeStr=T_M_Nm_Float32  PortDimensions=240
  ICARve_d_SignalTStamp : Outport  Port=37  OutDataTypeStr=UInt16
  wires:
  ICAR/26(ICARva_d_obj_MtnStat) -> ICARva_d_obj_MotionStatus/1
  ICAR/36(ICARva_g_ObjVelVarXYPre) -> ICARva_g_ObjVelVarXYPre/1
  IMAPve_d_PEPS_Door_Lock_Req/1 -> ICAR/41(IMAPve_d_PEPS_Door_Lock_Req)
  IMAPve_g_R0_C2_Back/1 -> ICAR/300(IMAPve_g_R0_C2_Back)
  ICAR/34(ICARva_g_ObjVelVarXPre) -> ICARva_g_ObjVelVarXPre/1
  IMAPve_d_ESC_Brake_Failsafe/1 -> ICAR/101(IMAPve_d_ESC_Brake_Failsafe)
  IMAPve_d_R0_LC/1 -> ICAR/266(IMAPve_d_R0_LC)
  IMAPva_d_obj_lane/1 -> ICAR/228(IMAPva_d_obj_lane)
  IMAPve_g_R0_Range_FR_Pred/1 -> ICAR/306(IMAPve_g_R0_Range_FR_Pred)
  IMAPve_g_ORI_R0_TLC/1 -> ICAR/190(IMAPve_g_ORI_R0_TLC)
  IMAPve_g_L0_C2_FR_Pred/1 -> ICAR/296(IMAPve_g_L0_C2_FR_Pred)
  IMAPve_g_R0_C2_FR_Pred/1 -> ICAR/305(IMAPve_g_R0_C2_FR_Pred)
  ICAR/35(ICARva_g_ObjVelVarYPre) -> ICARva_g_ObjVelVarYPre/1
  ICAR/3(ICARva_g_obj_pos_x) -> ICARva_g_obj_pos_x/1
  IMAPve_d_TBOX_LocalTime_Valid/1 -> ICAR/139(IMAPve_d_TBOX_LocalTime_Valid)
  ICAR/29(ICARva_g_ObjVarXPre) -> ICARva_g_ObjVarXPre/1
  ICAR/32(ICARva_g_ObjVelXPre) -> ICARva_g_ObjVelXPre/1
  IMAPve_g_EMS_Actual_FlwT/1 -> ICAR/51(IMAPve_g_EMS_Actual_FlwT)
  ICAR/7(ICARva_g_obj_acc_x) -> ICARva_g_obj_acc_x/1
  IMAPve_g_ESC_RR_WhlSpd/1 -> ICAR/88(IMAPve_g_ESC_RR_WhlSpd)
  IMAPva_g_obj_pos_y/1 -> ICAR/213(IMAPva_g_obj_pos_y)
  ICAR/25(ICARva_d_obj_BrkLi) -> ICARva_d_obj_BrakeLight/1
  IMAPve_d_LR_Radar_Status/1 -> ICAR/206(IMAPve_d_LR_Radar_Status)
  ICAR/27(ICARva_g_ObjXPre) -> ICARva_g_ObjXPre/1
  IMAPve_g_R0_C1_Back/1 -> ICAR/299(IMAPve_g_R0_C1_Back)
  ICAR/18(ICARva_d_obj_class) -> ICARva_d_obj_class/1
  ICAR/37(ICARve_d_SignalTStamp) -> ICARve_d_SignalTStamp/1
  ICAR/28(ICARva_g_ObjYPre) -> ICARva_g_ObjYPre/1
  IMAPve_g_R1_C0_Back/1 -> ICAR/316(IMAPve_g_R1_C0_Back)
  IMAPve_d_R1_LC/1 -> ICAR/288(IMAPve_d_R1_LC)
  IMAPve_g_R0_Confidence/1 -> ICAR/263(IMAPve_g_R0_Confidence)
  IMAPve_d_TCU_DCT_Clutch_State/1 -> ICAR/96(IMAPve_d_TCU_DCT_Clutch_State)
  IMAPve_d_EPS_TrqLim_State/1 -> ICAR/13(IMAPve_d_EPS_TrqLim_State)
  IMAPve_d_EPB_Warn_Req/1 -> ICAR/121(IMAPve_d_EPB_Warn_Req)
  IMAPve_d_ORI_Lane_Valid/1 -> ICAR/160(IMAPve_d_ORI_Lane_Valid)
  IMAPve_d_TBOX_LocalTimeMin/1 -> ICAR/137(IMAPve_d_TBOX_LocalTimeMin)
  ICAR/23(ICARva_d_obj_age) -> ICARva_d_obj_age/1
  ICAR/11(ICARva_g_obj_pos_var_xy) -> ICARva_g_obj_pos_var_xy/1
  IMAPve_d_L0_Q/1 -> ICAR/250(IMAPve_d_L0_Q)
  IMAPva_g_obj_vel_var_xy/1 -> ICAR/223(IMAPva_g_obj_vel_var_xy)
  IMAPve_g_R0_C0/1 -> ICAR/256(IMAPve_g_R0_C0)
  IMAPve_g_ORI_L1_C2/1 -> ICAR/174(IMAPve_g_ORI_L1_C2)
  ICAR/22(ICARva_g_obj_con) -> ICARva_g_obj_con/1
  IMAPve_g_EPS_PowerCon/1 -> ICAR/128(IMAPve_g_EPS_PowerCon)
  IMAPve_g_R1_C2_FR_Pred/1 -> ICAR/323(IMAPve_g_R1_C2_FR_Pred)
  ICAR/2(ICARva_d_obj_id) -> ICARva_d_obj_id/1
  IMAPve_g_L0_C0_Back/1 -> ICAR/289(IMAPve_g_L0_C0_Back)
  ICAR/24(ICARva_d_obj_TurnLi) -> ICARva_d_obj_TurnLight/1
  ICAR/17(ICARva_d_obj_fusion_type) -> ICARva_d_obj_fusion_type/1
  IMAPve_g_ORI_L0_C3/1 -> ICAR/163(IMAPve_g_ORI_L0_C3)
  ICAR/21(ICARve_d_obj_cam_asso_id) -> ICARve_d_obj_cam_asso_id/1
  ICAR/5(ICARva_g_obj_vel_x) -> ICARva_g_obj_vel_x/1
  ICABva_g_VehParameter/1 -> ICAR/4(ICABva_g_VehParameter)
  ICAR/19(ICARva_d_obj_lane) -> ICARva_d_obj_lane/1
  IMAPve_g_R1_C0/1 -> ICAR/278(IMAPve_g_R1_C0)
  IMAPve_d_ESC_ACC_Status/1 -> ICAR/105(IMAPve_d_ESC_ACC_Status)
  IMAPve_d_ORI_L0_LC/1 -> ICAR/172(IMAPve_d_ORI_L0_LC)
  IMAPve_d_ORI_Obj_Num/1 -> ICAR/149(IMAPve_d_ORI_Obj_Num)
  IMAPve_d_R0_Q/1 -> ICAR/261(IMAPve_d_R0_Q)
  IMAPve_d_Radar_State/1 -> ICAR/141(IMAPve_d_Radar_State)
  IMAPve_g_ORI_L1_C1/1 -> ICAR/175(IMAPve_g_ORI_L1_C1)
  IMAPve_g_L0_VR/1 -> ICAR/249(IMAPve_g_L0_VR)
  ICAR/14(ICARva_g_obj_vel_var_xy) -> ICARva_g_obj_vel_var_xy/1
  IMAPve_g_R1_C2_Back/1 -> ICAR/318(IMAPve_g_R1_C2_Back)
  IMAPve_d_BCM_RR_Door_State/1 -> ICAR/37(IMAPve_d_BCM_RR_Door_State)
  IMAPve_g_EMS_Engine_Speed/1 -> ICAR/58(IMAPve_g_EMS_Engine_Speed)
  IMAPve_d_ORI_R1_LC/1 -> ICAR/202(IMAPve_d_ORI_R1_LC)
  ICAR/8(ICARva_g_obj_acc_y) -> ICARva_g_obj_acc_y/1
  IMAPve_g_L1_C0/1 -> ICAR/267(IMAPve_g_L1_C0)
  IMAPve_d_TCU_Actual_Gear/1 -> ICAR/60(IMAPve_d_TCU_Actual_Gear)
  IMAPve_g_R1_C3/1 -> ICAR/281(IMAPve_g_R1_C3)
  IMAPve_g_L0_C3/1 -> ICAR/248(IMAPve_g_L0_C3)
  ICAR/1(ICARva_d_obj_Num) -> ICARva_d_obj_Num/1
  IMAPve_d_Radar_Status/1 -> ICAR/328(IMAPve_d_Radar_Status)
  IMAPva_g_obj_width/1 -> ICAR/224(IMAPva_g_obj_width)
  IMAPve_g_L0_C1_FR_Pred/1 -> ICAR/295(IMAPve_g_L0_C1_FR_Pred)
  IMAPve_d_ConsArea/1 -> ICAR/244(IMAPve_d_ConsArea)
  IMAPve_g_L1_C3/1 -> ICAR/270(IMAPve_g_L1_C3)
  IMAPve_g_R1_C0_FR_Pred/1 -> ICAR/321(IMAPve_g_R1_C0_FR_Pred)
  IMAPve_d_GW_Brake_Only_Req/1 -> ICAR/112(IMAPve_d_GW_Brake_Only_Req)
  IMAPve_d_EMS_ACC_CtlAvail/1 -> ICAR/114(IMAPve_d_EMS_ACC_CtlAvail)
  IMAPve_d_ORI_L1_LC/1 -> ICAR/182(IMAPve_d_ORI_L1_LC)
  IMAPve_g_L1_VR/1 -> ICAR/271(IMAPve_g_L1_VR)
  IMAPve_g_R1_Range_Back/1 -> ICAR/320(IMAPve_g_R1_Range_Back)
  IMAPve_g_R0_TLC/1 -> ICAR/265(IMAPve_g_R0_TLC)
  IMAPve_g_ORI_L0_C1/1 -> ICAR/165(IMAPve_g_ORI_L0_C1)
  IMAPve_g_R1_C1_FR_Pred/1 -> ICAR/322(IMAPve_g_R1_C1_FR_Pred)
  IMAPve_d_ESC_RL_WhlSpd_Fault/1 -> ICAR/87(IMAPve_d_ESC_RL_WhlSpd_Fault)
  IMAPve_d_Sign_ISA_Value/1 -> ICAR/325(IMAPve_d_Sign_ISA_Value)
  IMAPve_g_R1_C2/1 -> ICAR/280(IMAPve_g_R1_C2)
  IMAPve_d_TSR_Sign_Type/1 -> ICAR/326(IMAPve_d_TSR_Sign_Type)
  IMAPve_g_R1_Range_FR_Pred/1 -> ICAR/324(IMAPve_g_R1_Range_FR_Pred)
  IMAPve_g_L1_Range_FR_Pred/1 -> ICAR/315(IMAPve_g_L1_Range_FR_Pred)
  ICAR/10(ICARva_g_obj_pos_var_y) -> ICARva_g_obj_pos_var_y/1
  IMAPve_g_ORI_L0_VR/1 -> ICAR/169(IMAPve_g_ORI_L0_VR)
  IMAPve_d_BCM_Opening_State/1 -> ICAR/33(IMAPve_d_BCM_Opening_State)
  IMAPve_g_L1_C1_FR_Pred/1 -> ICAR/313(IMAPve_g_L1_C1_FR_Pred)
  IMAPve_g_FAPA_State/1 -> ICAR/146(IMAPve_g_FAPA_State)
  IMAPve_d_ESC_RR_WheelPulVal/1 -> ICAR/81(IMAPve_d_ESC_RR_WheelPulVal)
  IMAPve_d_TBOX_LocalTimeD/1 -> ICAR/135(IMAPve_d_TBOX_LocalTimeD)
  IMAPve_d_ESC_EBD_AlarmSig/1 -> ICAR/129(IMAPve_d_ESC_EBD_AlarmSig)
  IMAPve_g_L1_C2_FR_Pred/1 -> ICAR/314(IMAPve_g_L1_C2_FR_Pred)
  IMAPve_g_L0_C2/1 -> ICAR/247(IMAPve_g_L0_C2)
  IMAPve_g_L1_Range_Back/1 -> ICAR/311(IMAPve_g_L1_Range_Back)
  IMAPve_g_L0_C3_Back/1 -> ICAR/292(IMAPve_g_L0_C3_Back)
  IMAPve_g_L0_C2_Back/1 -> ICAR/291(IMAPve_g_L0_C2_Back)
  IMAPve_g_R0_C1/1 -> ICAR/257(IMAPve_g_R0_C1)
  IMAPva_g_obj_con/1 -> ICAR/231(IMAPva_g_obj_con)
  IMAPve_d_LF_Radar_Status/1 -> ICAR/204(IMAPve_d_LF_Radar_Status)
  IMAPve_g_R1_Confidence/1 -> ICAR/285(IMAPve_g_R1_Confidence)
  IMAPve_g_EMS_Actual_IndT/1 -> ICAR/52(IMAPve_g_EMS_Actual_IndT)
  IMAPve_g_ORI_R1_W/1 -> ICAR/201(IMAPve_g_ORI_R1_W)
  IMAPve_d_ESC_LatAcc_Valid/1 -> ICAR/16(IMAPve_d_ESC_LatAcc_Valid)
  IMAPve_g_L1_W/1 -> ICAR/275(IMAPve_g_L1_W)
  IMAPve_d_ORI_L0_Q/1 -> ICAR/167(IMAPve_d_ORI_L0_Q)
  IMAPve_g_L1_Confidence/1 -> ICAR/274(IMAPve_g_L1_Confidence)
  IMAPve_g_L1_TLC/1 -> ICAR/276(IMAPve_g_L1_TLC)
  ICAR/31(ICARva_g_ObjVarXYPre) -> ICARva_g_ObjVarXYPre/1
  IMAPve_d_L1_LC/1 -> ICAR/277(IMAPve_d_L1_LC)
  IMAPve_g_R0_C2/1 -> ICAR/258(IMAPve_g_R0_C2)
  IMAPve_d_R1_Q/1 -> ICAR/283(IMAPve_d_R1_Q)
  IMAPve_g_ORI_R1_TLC/1 -> ICAR/200(IMAPve_g_ORI_R1_TLC)
  IMAPve_d_BCM_LowBeam_State/1 -> ICAR/117(IMAPve_d_BCM_LowBeam_State)
  IMAPve_d_ORI_L1_Q/1 -> ICAR/177(IMAPve_d_ORI_L1_Q)
  IMAPve_d_EPS_Warning_State/1 -> ICAR/127(IMAPve_d_EPS_Warning_State)
  IMAPve_d_L1_Type/1 -> ICAR/273(IMAPve_d_L1_Type)
  IMAPve_d_Sensor_Status/1 -> ICAR/203(IMAPve_d_Sensor_Status)
  IMAPve_g_R0_C0_FR_Pred/1 -> ICAR/303(IMAPve_g_R0_C0_FR_Pred)
  IMAPve_d_L1_Q/1 -> ICAR/272(IMAPve_d_L1_Q)
  IMAPve_g_ORI_L0_TLC/1 -> ICAR/170(IMAPve_g_ORI_L0_TLC)
  IMAPve_d_Road_Type/1 -> ICAR/243(IMAPve_d_Road_Type)
  IMAPve_g_L1_C2/1 -> ICAR/269(IMAPve_g_L1_C2)
  IMAPve_d_Lane_Valid/1 -> ICAR/242(IMAPve_d_Lane_Valid)
  IMAPve_d_ORI_R0_LT/1 -> ICAR/188(IMAPve_d_ORI_R0_LT)
  IMAPve_d_BCM_LF_Door_State/1 -> ICAR/35(IMAPve_d_BCM_LF_Door_State)
  IMAPve_d_L0_LC/1 -> ICAR/255(IMAPve_d_L0_LC)
  IMAPve_g_L0_TLC/1 -> ICAR/254(IMAPve_g_L0_TLC)
  IMAPve_d_Outside_Temp/1 -> ICAR/147(IMAPve_d_Outside_Temp)
  IMAPve_g_R1_W/1 -> ICAR/286(IMAPve_g_R1_W)
  IMAPve_g_L0_Confidence/1 -> ICAR/252(IMAPve_g_L0_Confidence)
  IMAPve_g_R1_C3_Back/1 -> ICAR/319(IMAPve_g_R1_C3_Back)
  IMAPve_g_ESC_Brake_Press/1 -> ICAR/23(IMAPve_g_ESC_Brake_Press)
  IMAPve_g_L0_C0/1 -> ICAR/245(IMAPve_g_L0_C0)
  IMAPve_g_R1_C1_Back/1 -> ICAR/317(IMAPve_g_R1_C1_Back)
  IMAPve_g_ORI_L0_C0/1 -> ICAR/166(IMAPve_g_ORI_L0_C0)
  IMAPve_d_Radar_Detective_Req/1 -> ICAR/131(IMAPve_d_Radar_Detective_Req)
  IMAPve_g_ORI_R1_VR/1 -> ICAR/199(IMAPve_g_ORI_R1_VR)
  IMAPva_d_obj_status/1 -> ICAR/229(IMAPva_d_obj_status)
  IMAPve_g_ORI_L1_C3/1 -> ICAR/173(IMAPve_g_ORI_L1_C3)
  IMAPva_d_obj_MotionStatus/1 -> ICAR/235(IMAPva_d_obj_MotionStatus)
  IMAPve_g_R1_TLC/1 -> ICAR/287(IMAPve_g_R1_TLC)
  IMAPve_g_L1_C0_FR_Pred/1 -> ICAR/312(IMAPve_g_L1_C0_FR_Pred)
  IMAPva_g_obj_age/1 -> ICAR/232(IMAPva_g_obj_age)
  IMAPva_d_obj_TurnLight/1 -> ICAR/233(IMAPva_d_obj_TurnLight)
  ICAR/6(ICARva_g_obj_vel_y) -> ICARva_g_obj_vel_y/1
  IMAPve_d_ESC_Hold_State/1 -> ICAR/125(IMAPve_d_ESC_Hold_State)
  ICAR/9(ICARva_g_obj_pos_var_x) -> ICARva_g_obj_pos_var_x/1
  IMAPva_d_ORI_Obj_Lane/1 -> ICAR/155(IMAPva_d_ORI_Obj_Lane)
  IMAPve_d_ACU_Passenger_Belt/1 -> ICAR/113(IMAPve_d_ACU_Passenger_Belt)
  IMAPve_g_ORI_R0_C1/1 -> ICAR/185(IMAPve_g_ORI_R0_C1)
  IMAPva_d_obj_fusion_type/1 -> ICAR/226(IMAPva_d_obj_fusion_type)
  IMAPva_g_obj_vel_var_y/1 -> ICAR/222(IMAPva_g_obj_vel_var_y)
  IMAPve_g_ESC_VehSpd/1 -> ICAR/20(IMAPve_g_ESC_VehSpd)
  IMAPva_g_obj_vel_x/1 -> ICAR/214(IMAPva_g_obj_vel_x)
  IMAPva_g_ORI_Obj_RAngle/1 -> ICAR/157(IMAPva_g_ORI_Obj_RAngle)
  IMAPva_d_obj_ALC/1 -> ICAR/239(IMAPva_d_obj_ALC)
  IMAPve_d_R0_Type/1 -> ICAR/262(IMAPve_d_R0_Type)
  IMAPve_g_ESC_Static_Slope/1 -> ICAR/24(IMAPve_g_ESC_Static_Slope)
  IMAPve_d_RR_Radar_Status/1 -> ICAR/207(IMAPve_d_RR_Radar_Status)
  IMAPve_g_Fusion_Time_Stamp/1 -> ICAR/209(IMAPve_g_Fusion_Time_Stamp)
  ICAR/20(ICARva_d_obj_status) -> ICARva_d_obj_status/1
  IMAPva_g_obj_vel_var_x/1 -> ICAR/221(IMAPva_g_obj_vel_var_x)
  IMAPva_g_obj_pos_var_xy/1 -> ICAR/220(IMAPva_g_obj_pos_var_xy)
  IMAPva_d_obj_id/1 -> ICAR/211(IMAPva_d_obj_id)
  IMAPve_d_Camera_Signal_Fault/1 -> ICAR/327(IMAPve_d_Camera_Signal_Fault)
  IMAPve_g_ESC_YawRate/1 -> ICAR/17(IMAPve_g_ESC_YawRate)
  IMAPve_g_EMS_Pot_WhlT_Min/1 -> ICAR/45(IMAPve_g_EMS_Pot_WhlT_Min)
  IMAPve_d_ESC_ABS_AlarmSig/1 -> ICAR/77(IMAPve_d_ESC_ABS_AlarmSig)
  IMAPva_g_obj_acc_y/1 -> ICAR/217(IMAPva_g_obj_acc_y)
  IMAPve_d_ORI_R0_Q/1 -> ICAR/187(IMAPve_d_ORI_R0_Q)
  IMAPve_d_obj_Num/1 -> ICAR/210(IMAPve_d_obj_Num)
  IMAPve_d_R1_Type/1 -> ICAR/284(IMAPve_d_R1_Type)
  IMAPva_g_obj_pos_var_y/1 -> ICAR/219(IMAPva_g_obj_pos_var_y)
  IMAPve_g_ORI_R0_C0/1 -> ICAR/186(IMAPve_g_ORI_R0_C0)
  IMAPve_d_TBOX_LocalTimeY/1 -> ICAR/133(IMAPve_d_TBOX_LocalTimeY)
  IMAPve_d_ORI_Lane_ConsArea/1 -> ICAR/161(IMAPve_d_ORI_Lane_ConsArea)
  IMAPve_g_EPS_LKA_Current/1 -> ICAR/14(IMAPve_g_EPS_LKA_Current)
  IMAPve_g_EMS_MinTWhl/1 -> ICAR/49(IMAPve_g_EMS_MinTWhl)
  IMAPva_g_ORI_Obj_LongDis/1 -> ICAR/154(IMAPva_g_ORI_Obj_LongDis)
  IMAPve_g_ORI_R0_C2/1 -> ICAR/184(IMAPve_g_ORI_R0_C2)
  IMAPve_d_EMS_ACC_Effective/1 -> ICAR/108(IMAPve_d_EMS_ACC_Effective)
  IMAPve_d_ORI_R1_LT/1 -> ICAR/198(IMAPve_d_ORI_R1_LT)
  IMAPve_d_ORI_R1_Q/1 -> ICAR/197(IMAPve_d_ORI_R1_Q)
  IMAPve_g_L0_W/1 -> ICAR/253(IMAPve_g_L0_W)
  ICAR/30(ICARva_g_ObjVarYPre) -> ICARva_g_ObjVarYPre/1
  IMAPve_g_ORI_R0_W/1 -> ICAR/191(IMAPve_g_ORI_R0_W)
  IMAPve_g_ORI_R0_C3/1 -> ICAR/183(IMAPve_g_ORI_R0_C3)
  IMAPve_d_ORI_Lane_RoadType/1 -> ICAR/162(IMAPve_d_ORI_Lane_RoadType)
  IMAPve_d_ESC_FR_Wheel_Pulse/1 -> ICAR/91(IMAPve_d_ESC_FR_Wheel_Pulse)
  IMAPve_d_EPS_Trq_State/1 -> ICAR/10(IMAPve_d_EPS_Trq_State)
  ICAR/15(ICARva_g_obj_width) -> ICARva_g_obj_width/1
  IMAPve_g_ORI_L1_VR/1 -> ICAR/179(IMAPve_g_ORI_L1_VR)
  IMAPve_d_EMS_ACC_Inhibited/1 -> ICAR/115(IMAPve_d_EMS_ACC_Inhibited)
  IMAPve_d_BCM_FrontWiper_State/1 -> ICAR/109(IMAPve_d_BCM_FrontWiper_State)
  IMAPva_g_ORI_Obj_LAngle/1 -> ICAR/156(IMAPva_g_ORI_Obj_LAngle)
  IMAPva_g_ORI_Obj_RelVel/1 -> ICAR/153(IMAPva_g_ORI_Obj_RelVel)
  IMAPve_g_ORI_R1_C3/1 -> ICAR/193(IMAPve_g_ORI_R1_C3)
  IMAPve_d_RF_Radar_Status/1 -> ICAR/205(IMAPve_d_RF_Radar_Status)
  IMAPve_d_ORI_L1_Type/1 -> ICAR/178(IMAPve_d_ORI_L1_Type)
  IMAPve_g_ORI_L1_TLC/1 -> ICAR/180(IMAPve_g_ORI_L1_TLC)
  IMAPve_g_ORI_L1_C0/1 -> ICAR/176(IMAPve_g_ORI_L1_C0)
  IMAPve_g_L0_C1_Back/1 -> ICAR/290(IMAPve_g_L0_C1_Back)
  IMAPva_g_ORI_Probability/1 -> ICAR/150(IMAPva_g_ORI_Probability)
  IMAPve_d_ACC_Desired_Headway/1 -> ICAR/142(IMAPve_d_ACC_Desired_Headway)
  IMAPve_g_L0_C1/1 -> ICAR/246(IMAPve_g_L0_C1)
  IMAPve_g_EMS_Pot_WhlT_Max/1 -> ICAR/44(IMAPve_g_EMS_Pot_WhlT_Max)
  IMAPve_g_ORI_L1_W/1 -> ICAR/181(IMAPve_g_ORI_L1_W)
  IMAPva_d_ORI_Obj_Class/1 -> ICAR/151(IMAPva_d_ORI_Obj_Class)
  IMAPve_d_ESC_FR_WheelPulVal/1 -> ICAR/79(IMAPve_d_ESC_FR_WheelPulVal)
  IMAPve_g_BCM_Battery_Voltage/1 -> ICAR/132(IMAPve_g_BCM_Battery_Voltage)
  IMAPve_d_Time_System_Clock/1 -> ICAR/143(IMAPve_d_Time_System_Clock)
  IMAPve_d_ESC_AVH_Status/1 -> ICAR/130(IMAPve_d_ESC_AVH_Status)
  IMAPve_d_EPB_Switch_Valid/1 -> ICAR/123(IMAPve_d_EPB_Switch_Valid)
  IMAPve_g_ORI_L0_C2/1 -> ICAR/164(IMAPve_g_ORI_L0_C2)
  IMAPve_d_EPB_Status/1 -> ICAR/119(IMAPve_d_EPB_Status)
  IMAPve_d_ESC_RL_WheelPulVal/1 -> ICAR/80(IMAPve_d_ESC_RL_WheelPulVal)
  IMAPva_d_obj_class/1 -> ICAR/227(IMAPva_d_obj_class)
  IMAPve_d_ORI_CIPV_ID/1 -> ICAR/148(IMAPve_d_ORI_CIPV_ID)
  IMAPve_d_BCM_BrakeLamp_State/1 -> ICAR/111(IMAPve_d_BCM_BrakeLamp_State)
  IMAPve_d_EPS_Error_State/1 -> ICAR/9(IMAPve_d_EPS_Error_State)
  IMAPve_d_BCM_HighBeam_State/1 -> ICAR/118(IMAPve_d_BCM_HighBeam_State)
  IMAPve_d_EPS_Steer_Hold_State/1 -> ICAR/126(IMAPve_d_EPS_Steer_Hold_State)
  IMAPve_g_GW_IC_Odometer/1 -> ICAR/145(IMAPve_g_GW_IC_Odometer)
  IMAPve_g_ORI_R1_C1/1 -> ICAR/195(IMAPve_g_ORI_R1_C1)
  IMAPva_d_obj_ESA/1 -> ICAR/240(IMAPva_d_obj_ESA)
  IMAPve_g_ESC_UnYawRate/1 -> ICAR/19(IMAPve_g_ESC_UnYawRate)
  IMAPva_d_ORI_Obj_ID/1 -> ICAR/159(IMAPva_d_ORI_Obj_ID)
  IMAPve_d_ESC_Drive_Direction/1 -> ICAR/124(IMAPve_d_ESC_Drive_Direction)
  IMAPve_g_ESC_DySlope/1 -> ICAR/26(IMAPve_g_ESC_DySlope)
  IMAPve_d_ESC_AEB_Active/1 -> ICAR/104(IMAPve_d_ESC_AEB_Active)
  IMAPve_g_ORI_R1_C0/1 -> ICAR/196(IMAPve_g_ORI_R1_C0)
  IMAPve_d_TCU_AT_Failure/1 -> ICAR/94(IMAPve_d_TCU_AT_Failure)
  IMAPve_d_TBOX_LocalTimeM/1 -> ICAR/134(IMAPve_d_TBOX_LocalTimeM)
  IMAPve_d_ESC_RR_Wheel_Pulse/1 -> ICAR/93(IMAPve_d_ESC_RR_Wheel_Pulse)
  IMAPve_g_ESC_RL_WhlSpd/1 -> ICAR/86(IMAPve_g_ESC_RL_WhlSpd)
  IMAPve_d_ESC_RR_WhlSpd_Fault/1 -> ICAR/89(IMAPve_d_ESC_RR_WhlSpd_Fault)
  IMAPve_d_TCU_Select_ATMode/1 -> ICAR/98(IMAPve_d_TCU_Select_ATMode)
  IMAPve_d_EMS_Brake_Pedal/1 -> ICAR/116(IMAPve_d_EMS_Brake_Pedal)
  IMAPve_g_L1_C1/1 -> ICAR/268(IMAPve_g_L1_C1)
  IMAPve_d_ESC_RL_Wheel_Pulse/1 -> ICAR/92(IMAPve_d_ESC_RL_Wheel_Pulse)
  IMAPve_d_ESC_ACC_Active/1 -> ICAR/107(IMAPve_d_ESC_ACC_Active)
  IMAPve_d_ESC_AEB_Status/1 -> ICAR/102(IMAPve_d_ESC_AEB_Status)
  IMAPve_d_TCU_Shift_Valid/1 -> ICAR/95(IMAPve_d_TCU_Shift_Valid)
  IMAPve_d_BCM_CHMSL_Status/1 -> ICAR/110(IMAPve_d_BCM_CHMSL_Status)
  IMAPve_d_ESC_FL_Wheel_Pulse/1 -> ICAR/90(IMAPve_d_ESC_FL_Wheel_Pulse)
  IMAPve_d_EMS_Engine_Status/1 -> ICAR/99(IMAPve_d_EMS_Engine_Status)
  IMAPve_d_ESC_ESC_Active/1 -> ICAR/70(IMAPve_d_ESC_ESC_Active)
  IMAPve_d_ORI_R0_LC/1 -> ICAR/192(IMAPve_d_ORI_R0_LC)
  IMAPve_d_ESC_ACC_Available/1 -> ICAR/106(IMAPve_d_ESC_ACC_Available)
  IMAPve_d_ESC_MSR_Active/1 -> ICAR/71(IMAPve_d_ESC_MSR_Active)
  IMAPve_d_TCU_Gear_Engage/1 -> ICAR/97(IMAPve_d_TCU_Gear_Engage)
  IMAPve_d_ACU_Driver_Belt/1 -> ICAR/64(IMAPve_d_ACU_Driver_Belt)
  IMAPve_d_EPB_Switch_State/1 -> ICAR/122(IMAPve_d_EPB_Switch_State)
  IMAPve_d_SWS_Failure_Status/1 -> ICAR/66(IMAPve_d_SWS_Failure_Status)
  IMAPve_d_ESC_FL_WheelPulVal/1 -> ICAR/78(IMAPve_d_ESC_FL_WheelPulVal)
  IMAPve_d_ESC_AlarmSig/1 -> ICAR/68(IMAPve_d_ESC_AlarmSig)
  IMAPve_g_ESC_FR_WhlSpd/1 -> ICAR/84(IMAPve_g_ESC_FR_WhlSpd)
  IMAPve_d_SWS_Fault_Code/1 -> ICAR/65(IMAPve_d_SWS_Fault_Code)
  IMAPve_d_ESC_ABS_Valid/1 -> ICAR/76(IMAPve_d_ESC_ABS_Valid)
  IMAPve_d_Speed_Limit_Switch/1 -> ICAR/69(IMAPve_d_Speed_Limit_Switch)
  IMAPve_d_Signal_Time_Stamp/1 -> ICAR/144(IMAPve_d_Signal_Time_Stamp)
  IMAPve_d_ESC_VehSpd_Valid/1 -> ICAR/73(IMAPve_d_ESC_VehSpd_Valid)
  IMAPve_g_EMS_ACC_VirtualPedal/1 -> ICAR/54(IMAPve_g_EMS_ACC_VirtualPedal)
  IMAPve_d_TBOX_LocalTimeS/1 -> ICAR/138(IMAPve_d_TBOX_LocalTimeS)
  IMAPve_g_EMS_MaxTWhl/1 -> ICAR/47(IMAPve_g_EMS_MaxTWhl)
  IMAPve_g_EMS_MaxTWhl_Offset/1 -> ICAR/48(IMAPve_g_EMS_MaxTWhl_Offset)
  IMAPve_d_Brake_Pedal_Fault/1 -> ICAR/74(IMAPve_d_Brake_Pedal_Fault)
  IMAPve_d_BCM_Door_Lock_State/1 -> ICAR/42(IMAPve_d_BCM_Door_Lock_State)
  IMAPve_d_ESC_ABS_Active/1 -> ICAR/75(IMAPve_d_ESC_ABS_Active)
  IMAPve_d_ESC_Veh_Standstill/1 -> ICAR/59(IMAPve_d_ESC_Veh_Standstill)
  ICAR/12(ICARva_g_obj_vel_var_x) -> ICARva_g_obj_vel_var_x/1
  IMAPve_d_ESC_FL_WhlSpd_Fault/1 -> ICAR/83(IMAPve_d_ESC_FL_WhlSpd_Fault)
  IMAPva_d_ORI_Obj_Motion/1 -> ICAR/152(IMAPva_d_ORI_Obj_Motion)
  IMAPve_d_SCC_Left_SwitchSig/1 -> ICAR/39(IMAPve_d_SCC_Left_SwitchSig)
  IMAPve_d_EPB_Display_Req/1 -> ICAR/120(IMAPve_d_EPB_Display_Req)
  IMAPve_d_EMS_AccPedal_Fault/1 -> ICAR/55(IMAPve_d_EMS_AccPedal_Fault)
  IMAPve_d_BCM_Ignition_State/1 -> ICAR/63(IMAPve_d_BCM_Ignition_State)
  IMAPve_g_ORI_R0_VR/1 -> ICAR/189(IMAPve_g_ORI_R0_VR)
  IMAPve_g_EMS_RealPedal/1 -> ICAR/46(IMAPve_g_EMS_RealPedal)
  IMAPve_d_TCU_PRND_State/1 -> ICAR/62(IMAPve_d_TCU_PRND_State)
  IMAPve_g_EMS_Realize_TWhl/1 -> ICAR/53(IMAPve_g_EMS_Realize_TWhl)
  IMAPve_d_TPMS_Warn_Indicate/1 -> ICAR/140(IMAPve_d_TPMS_Warn_Indicate)
  IMAPve_d_ESC_Brake_Effort/1 -> ICAR/57(IMAPve_d_ESC_Brake_Effort)
  FDMMve_d_SignalTStamp/1 -> ICAR/3(FDMMve_d_SignalTStamp)
  IMAPve_g_ESC_LonAcc/1 -> ICAR/21(IMAPve_g_ESC_LonAcc)
  IMAPve_d_EPS_LKA_State/1 -> ICAR/7(IMAPve_d_EPS_LKA_State)
  IMAPve_d_EMS_ACC_Status/1 -> ICAR/43(IMAPve_d_EMS_ACC_Status)
  IMAPve_d_ORI_L0_Type/1 -> ICAR/168(IMAPve_d_ORI_L0_Type)
  IMAPve_d_BCM_Left_Light/1 -> ICAR/30(IMAPve_d_BCM_Left_Light)
  IMAPve_d_ESC_YawRate_Valid/1 -> ICAR/18(IMAPve_d_ESC_YawRate_Valid)
  IMAPve_g_SW_Angle/1 -> ICAR/27(IMAPve_g_SW_Angle)
  IMAPve_g_ESC_DySlope_Accuracy/1 -> ICAR/25(IMAPve_g_ESC_DySlope_Accuracy)
  IMAPve_d_ESC_OFF/1 -> ICAR/67(IMAPve_d_ESC_OFF)
  IMAPve_d_ESC_LonAcc_Valid/1 -> ICAR/22(IMAPve_d_ESC_LonAcc_Valid)
  IMAPve_d_EMS_Gearbox_CtlAvail/1 -> ICAR/100(IMAPve_d_EMS_Gearbox_CtlAvail)
  IMAPve_d_TBOX_LocalTimeH/1 -> ICAR/136(IMAPve_d_TBOX_LocalTimeH)
  IMAPve_d_BCM_LR_Door_State/1 -> ICAR/38(IMAPve_d_BCM_LR_Door_State)
  IMAPve_g_SW_Angle_Speed/1 -> ICAR/28(IMAPve_g_SW_Angle_Speed)
  IMAPve_d_BCM_HazardLamp/1 -> ICAR/29(IMAPve_d_BCM_HazardLamp)
  IMAPve_d_ESC_AEB_Available/1 -> ICAR/103(IMAPve_d_ESC_AEB_Available)
  IMAPve_d_BCM_RF_Door_State/1 -> ICAR/36(IMAPve_d_BCM_RF_Door_State)
  IMAPve_d_ESC_FR_WhlSpd_Fault/1 -> ICAR/85(IMAPve_d_ESC_FR_WhlSpd_Fault)
  IMAPve_d_ESC_BrakeLamp_Req/1 -> ICAR/32(IMAPve_d_ESC_BrakeLamp_Req)
  IMAPve_d_TCU_Target_Gear/1 -> ICAR/61(IMAPve_d_TCU_Target_Gear)
  IMAPve_g_EMS_Driver_Torque/1 -> ICAR/56(IMAPve_g_EMS_Driver_Torque)
  IMAPve_d_SAS_Trim_State/1 -> ICAR/12(IMAPve_d_SAS_Trim_State)
  IMAPve_d_Camera_Status/1 -> ICAR/329(IMAPve_d_Camera_Status)
  IMAPve_g_EMS_MinTWhl_Offset/1 -> ICAR/50(IMAPve_g_EMS_MinTWhl_Offset)
  ICABve_d_SignalTStamp/1 -> ICAR/6(ICABve_d_SignalTStamp)
  ICABva_g_FilterInfo/1 -> ICAR/5(ICABva_g_FilterInfo)
  FDMMve_d_IcaFcnConf/1 -> ICAR/2(FDMMve_d_IcaFcnConf)
  IMAPve_g_ORI_R1_C2/1 -> ICAR/194(IMAPve_g_ORI_R1_C2)
  IMAPva_d_obj_cam_asso_id/1 -> ICAR/230(IMAPva_d_obj_cam_asso_id)
  IMAPve_g_ESC_LatAcc/1 -> ICAR/15(IMAPve_g_ESC_LatAcc)
  IMAPve_g_L1_C2_Back/1 -> ICAR/309(IMAPve_g_L1_C2_Back)
  IMAPva_g_obj_acc_x/1 -> ICAR/216(IMAPva_g_obj_acc_x)
  IMAPve_g_R0_C0_Back/1 -> ICAR/298(IMAPve_g_R0_C0_Back)
  IMAPve_d_BCM_Trunk_State/1 -> ICAR/34(IMAPve_d_BCM_Trunk_State)
  IMAPve_g_R0_C1_FR_Pred/1 -> ICAR/304(IMAPve_g_R0_C1_FR_Pred)
  IMAPve_g_R0_VR/1 -> ICAR/260(IMAPve_g_R0_VR)
  IMAPve_g_R0_W/1 -> ICAR/264(IMAPve_g_R0_W)
  ICAR/33(ICARva_g_ObjVelYPre) -> ICARva_g_ObjVelYPre/1
  System_Clock/1 -> ICAR/1(System_Clock)
  IMAPva_g_obj_pos_x/1 -> ICAR/212(IMAPva_g_obj_pos_x)
  IMAPve_g_R1_VR/1 -> ICAR/282(IMAPve_g_R1_VR)
  IMAPve_g_R0_Range_Back/1 -> ICAR/302(IMAPve_g_R0_Range_Back)
  IMAPve_g_L1_C1_Back/1 -> ICAR/308(IMAPve_g_L1_C1_Back)
  IMAPve_d_BCM_Right_Light/1 -> ICAR/31(IMAPve_d_BCM_Right_Light)
  ICAR/13(ICARva_g_obj_vel_var_y) -> ICARva_g_obj_vel_var_y/1
  IMAPve_g_ORI_L0_W/1 -> ICAR/171(IMAPve_g_ORI_L0_W)
  IMAPve_g_L1_C0_Back/1 -> ICAR/307(IMAPve_g_L1_C0_Back)
  IMAPva_g_obj_length/1 -> ICAR/225(IMAPva_g_obj_length)
  IMAPva_g_obj_vel_y/1 -> ICAR/215(IMAPva_g_obj_vel_y)
  IMAPve_g_ESC_FL_WhlSpd/1 -> ICAR/82(IMAPve_g_ESC_FL_WhlSpd)
  IMAPve_d_L0_Type/1 -> ICAR/251(IMAPve_d_L0_Type)
  IMAPva_d_obj_ELK/1 -> ICAR/238(IMAPva_d_obj_ELK)
  IMAPva_d_obj_JA/1 -> ICAR/241(IMAPva_d_obj_JA)
  ICAR/16(ICARva_d_obj_length) -> ICARva_d_obj_length/1
  IMAPve_d_SCC_Right_SwitchSig/1 -> ICAR/40(IMAPve_d_SCC_Right_SwitchSig)
  IMAPve_d_ESC_TCS_Active/1 -> ICAR/72(IMAPve_d_ESC_TCS_Active)
  IMAPva_g_ORI_Obj_Width/1 -> ICAR/158(IMAPva_g_ORI_Obj_Width)
  IMAPve_g_R1_C1/1 -> ICAR/279(IMAPve_g_R1_C1)
  IMAPve_g_L0_Range_FR_Pred/1 -> ICAR/297(IMAPve_g_L0_Range_FR_Pred)
  IMAPve_g_L0_C0_FR_Pred/1 -> ICAR/294(IMAPve_g_L0_C0_FR_Pred)
  IMAPva_d_obj_AEB/1 -> ICAR/237(IMAPva_d_obj_AEB)
  ICAR/4(ICARva_g_obj_pos_y) -> ICARva_g_obj_pos_y/1
  IMAPve_d_SAS_Clb_State/1 -> ICAR/11(IMAPve_d_SAS_Clb_State)
  IMAPve_g_L0_Range_Back/1 -> ICAR/293(IMAPve_g_L0_Range_Back)
  IMAPva_d_obj_ACC/1 -> ICAR/236(IMAPva_d_obj_ACC)
  IMAPve_g_EPS_SW_Trq/1 -> ICAR/8(IMAPve_g_EPS_SW_Trq)
  IMAPve_g_L1_C3_Back/1 -> ICAR/310(IMAPve_g_L1_C3_Back)
  IMAPve_g_R0_C3/1 -> ICAR/259(IMAPve_g_R0_C3)
  IMAPva_d_obj_BrakeLight/1 -> ICAR/234(IMAPva_d_obj_BrakeLight)
  IMAPve_g_R0_C3_Back/1 -> ICAR/301(IMAPve_g_R0_C3_Back)
  IMAPva_g_obj_pos_var_x/1 -> ICAR/218(IMAPva_g_obj_pos_var_x)
  IMAPve_d_Fusion_Status/1 -> ICAR/208(IMAPve_d_Fusion_Status)
